simulink library "Solver_DS_SF"  (Simulink 7.1)
libraries: simulink x65
(part 2 of 2)

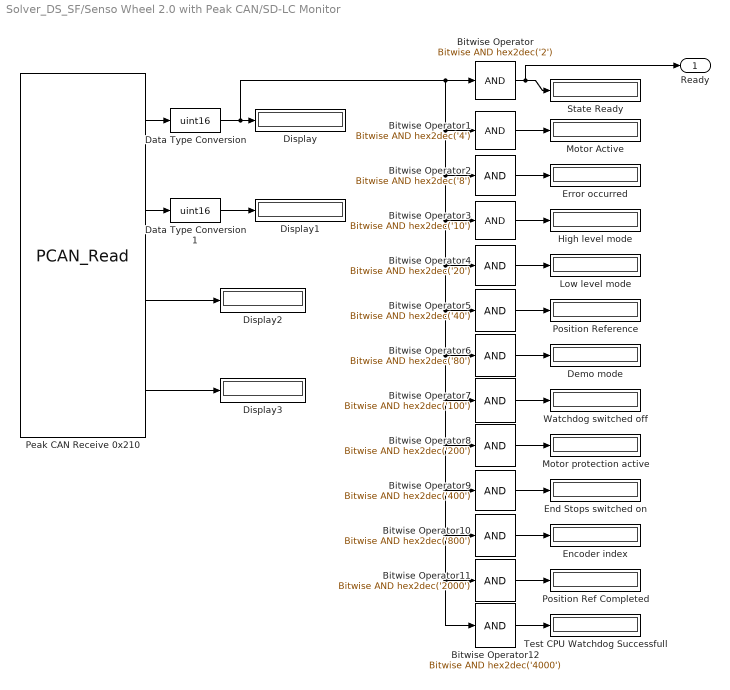
== system Solver_DS_SF/Senso Wheel 2.0 with Peak CAN/SD-LC Monitor ==
  Bitwise Operator : simulink/Logic and Bit Operations/Bitwise Operator  logicop=AND  UseBitMask=on  BitMask=hex2dec('2')  BitMaskRealWorld=Stored Integer
  Bitwise Operator1 : simulink/Logic and Bit Operations/Bitwise Operator  logicop=AND  UseBitMask=on  BitMask=hex2dec('4')  BitMaskRealWorld=Stored Integer
  Bitwise Operator10 : simulink/Logic and Bit Operations/Bitwise Operator  logicop=AND  UseBitMask=on  BitMask=hex2dec('800')  BitMaskRealWorld=Stored Integer
  Bitwise Operator11 : simulink/Logic and Bit Operations/Bitwise Operator  logicop=AND  UseBitMask=on  BitMask=hex2dec('2000')  BitMaskRealWorld=Stored Integer
  Bitwise Operator12 : simulink/Logic and Bit Operations/Bitwise Operator  logicop=AND  UseBitMask=on  BitMask=hex2dec('4000')  BitMaskRealWorld=Stored Integer
  Bitwise Operator2 : simulink/Logic and Bit Operations/Bitwise Operator  logicop=AND  UseBitMask=on  BitMask=hex2dec('8')  BitMaskRealWorld=Stored Integer
  Bitwise Operator3 : simulink/Logic and Bit Operations/Bitwise Operator  logicop=AND  UseBitMask=on  BitMask=hex2dec('10')  BitMaskRealWorld=Stored Integer
  Bitwise Operator4 : simulink/Logic and Bit Operations/Bitwise Operator  logicop=AND  UseBitMask=on  BitMask=hex2dec('20')  BitMaskRealWorld=Stored Integer
  Bitwise Operator5 : simulink/Logic and Bit Operations/Bitwise Operator  logicop=AND  UseBitMask=on  BitMask=hex2dec('40')  BitMaskRealWorld=Stored Integer
  Bitwise Operator6 : simulink/Logic and Bit Operations/Bitwise Operator  logicop=AND  UseBitMask=on  BitMask=hex2dec('80')  BitMaskRealWorld=Stored Integer
  Bitwise Operator7 : simulink/Logic and Bit Operations/Bitwise Operator  logicop=AND  UseBitMask=on  BitMask=hex2dec('100')  BitMaskRealWorld=Stored Integer
  Bitwise Operator8 : simulink/Logic and Bit Operations/Bitwise Operator  logicop=AND  UseBitMask=on  BitMask=hex2dec('200')  BitMaskRealWorld=Stored Integer
  Bitwise Operator9 : simulink/Logic and Bit Operations/Bitwise Operator  logicop=AND  UseBitMask=on  BitMask=hex2dec('400')  BitMaskRealWorld=Stored Integer
  Data Type Conversion : DataTypeConversion  OutDataTypeStr=uint16  OutDataTypeMode=uint16  RndMeth=Zero
  Data Type Conversion1 : DataTypeConversion  OutDataTypeStr=uint16  OutDataTypeMode=uint16  RndMeth=Zero
  Demo mode : Display
  Display{,1..3} (4 alike) : Display
  Encoder index : Display
  End Stops switched on : Display
  Error occurred : Display
  High level mode : Display
  Low level mode : Display
  Motor Active : Display
  Motor protection active : Display
  Peak CAN Receive 0x210 : S-Function  FunctionName=PCAN_Read  Parameters=id,TimeStep,nOut,bits_define  EnableBusSupport=off  mask{id=528, TimeStep=0.1, bits_define={[0:15],[16:31],[32:47],[48:63]}, portnames={'Status','Errors','End Stop Position','Encodeer Index Position'}}
      mask prompts: id "CAN ID"; TimeStep "Sample time"; bits_define "Bit defination (cell array):"; portnames "Port name (cell array):"
      mask init:
      | nOut=length(bits_define);
      | [bits_define]=formatbit(bits_define,portnames,1);
      | set_param(gcb, 'Parameters', ['id,TimeStep,nOut,bits_define']);
      mask Display: port_label('output',1,'Status ');port_label('output',2,'Errors ');port_label('output',3,'End Stop Position ');port_label('output',4,'Encodeer Index Position ');
  Position Ref Completed : Display
  Position Reference : Display
  State Ready : Display
  Test CPU Watchdog Successfull : Display
  Watchdog switched off : Display
  Ready : Outport  InitialOutput=0
  wires:
  Data Type Conversion/1 -> Display/1, Bitwise Operator7/1, Bitwise Operator8/1, Bitwise Operator9/1, Bitwise Operator10/1, Bitwise Operator11/1, Bitwise Operator12/1, Bitwise Operator6/1, Bitwise Operator5/1, Bitwise Operator4/1, Bitwise Operator3/1, Bitwise Operator2/1, Bitwise Operator1/1, Bitwise Operator/1
  Bitwise Operator12/1 -> Test CPU Watchdog Successfull/1
  Bitwise Operator11/1 -> Position Ref Completed/1
  Bitwise Operator10/1 -> Encoder index/1
  Bitwise Operator9/1 -> End Stops switched on/1
  Bitwise Operator8/1 -> Motor protection active/1
  Bitwise Operator7/1 -> Watchdog switched off/1
  Bitwise Operator6/1 -> Demo mode/1
  Bitwise Operator5/1 -> Position Reference/1
  Bitwise Operator4/1 -> Low level mode/1
  Bitwise Operator3/1 -> High level mode/1
  Bitwise Operator2/1 -> Error occurred/1
  Bitwise Operator1/1 -> Motor Active/1
  Bitwise Operator/1 -> State Ready/1, Ready/1
  Data Type Conversion1/1 -> Display1/1
  Peak CAN Receive 0x210/4 -> Display3/1
  Peak CAN Receive 0x210/3 -> Display2/1
  Peak CAN Receive 0x210/2 -> Data Type Conversion1/1
  Peak CAN Receive 0x210/1 -> Data Type Conversion/1

== system Solver_DS_SF/Senso Wheel 2.0 with Peak CAN/Triggered Subsystem ==
  Trigger : TriggerPort
  Constant3 : Constant  OutDataTypeStr=uint8  OutDataTypeMode=uint8
  Ready : Outport  InitialOutput=0
  wires:
  Constant3/1 -> Ready/1

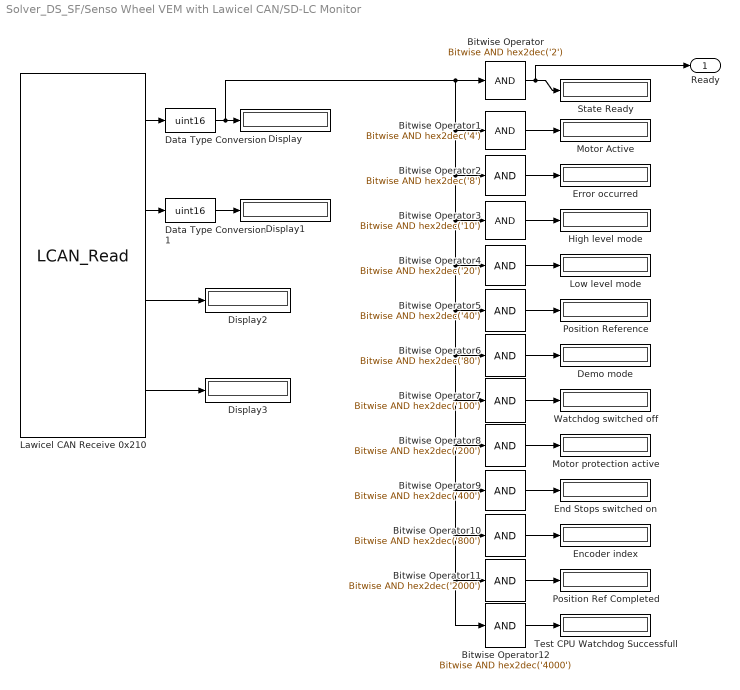
== system Solver_DS_SF/Senso Wheel VEM with Lawicel CAN/SD-LC Monitor ==
  Bitwise Operator : simulink/Logic and Bit Operations/Bitwise Operator  logicop=AND  UseBitMask=on  BitMask=hex2dec('2')  BitMaskRealWorld=Stored Integer
  Bitwise Operator1 : simulink/Logic and Bit Operations/Bitwise Operator  logicop=AND  UseBitMask=on  BitMask=hex2dec('4')  BitMaskRealWorld=Stored Integer
  Bitwise Operator10 : simulink/Logic and Bit Operations/Bitwise Operator  logicop=AND  UseBitMask=on  BitMask=hex2dec('800')  BitMaskRealWorld=Stored Integer
  Bitwise Operator11 : simulink/Logic and Bit Operations/Bitwise Operator  logicop=AND  UseBitMask=on  BitMask=hex2dec('2000')  BitMaskRealWorld=Stored Integer
  Bitwise Operator12 : simulink/Logic and Bit Operations/Bitwise Operator  logicop=AND  UseBitMask=on  BitMask=hex2dec('4000')  BitMaskRealWorld=Stored Integer
  Bitwise Operator2 : simulink/Logic and Bit Operations/Bitwise Operator  logicop=AND  UseBitMask=on  BitMask=hex2dec('8')  BitMaskRealWorld=Stored Integer
  Bitwise Operator3 : simulink/Logic and Bit Operations/Bitwise Operator  logicop=AND  UseBitMask=on  BitMask=hex2dec('10')  BitMaskRealWorld=Stored Integer
  Bitwise Operator4 : simulink/Logic and Bit Operations/Bitwise Operator  logicop=AND  UseBitMask=on  BitMask=hex2dec('20')  BitMaskRealWorld=Stored Integer
  Bitwise Operator5 : simulink/Logic and Bit Operations/Bitwise Operator  logicop=AND  UseBitMask=on  BitMask=hex2dec('40')  BitMaskRealWorld=Stored Integer
  Bitwise Operator6 : simulink/Logic and Bit Operations/Bitwise Operator  logicop=AND  UseBitMask=on  BitMask=hex2dec('80')  BitMaskRealWorld=Stored Integer
  Bitwise Operator7 : simulink/Logic and Bit Operations/Bitwise Operator  logicop=AND  UseBitMask=on  BitMask=hex2dec('100')  BitMaskRealWorld=Stored Integer
  Bitwise Operator8 : simulink/Logic and Bit Operations/Bitwise Operator  logicop=AND  UseBitMask=on  BitMask=hex2dec('200')  BitMaskRealWorld=Stored Integer
  Bitwise Operator9 : simulink/Logic and Bit Operations/Bitwise Operator  logicop=AND  UseBitMask=on  BitMask=hex2dec('400')  BitMaskRealWorld=Stored Integer
  Data Type Conversion : DataTypeConversion  OutDataTypeStr=uint16  OutDataTypeMode=uint16  RndMeth=Zero
  Data Type Conversion1 : DataTypeConversion  OutDataTypeStr=uint16  OutDataTypeMode=uint16  RndMeth=Zero
  Demo mode : Display
  Display{,1..3} (4 alike) : Display
  Encoder index : Display
  End Stops switched on : Display
  Error occurred : Display
  High level mode : Display
  Lawicel CAN Receive 0x210 : S-Function  FunctionName=LCAN_Read  Parameters=1,CAN_MODE,id,TimeStep,nOut,bits_define  EnableBusSupport=off  mask{adapter=CAN1, CAN_MODE=Standard (11-bit), id=528, TimeStep=0.1, bits_define={[0:15],[16:31],[32:47],[48:63]}, portnames={'Status','Errors','End Stop Position','Encodeer Index Position'}}
      mask prompts: adapter "CAN adapter"; CAN_MODE "CAN identifier range:"; id "CAN ID"; TimeStep "Sample time"; bits_define "Bit defination (cell array):"; portnames "Port name (cell array):"
      mask init:
      | nOut=length(bits_define);
      | [bits_define]=formatbit(bits_define,portnames,1);
      | set_param(gcb, 'Parameters', [adapter(4) ',CAN_MODE,id,TimeStep,nOut,bits_define']);
      mask StyleString: popup(CAN1|CAN2|CAN3|CAN4),popup(Standard (11-bit)|Extended (29-bit)),edit,edit,edit,edit
      mask Display: port_label('output',1,'Status ');port_label('output',2,'Errors ');port_label('output',3,'End Stop Position ');port_label('output',4,'Encodeer Index Position ');
  Low level mode : Display
  Motor Active : Display
  Motor protection active : Display
  Position Ref Completed : Display
  Position Reference : Display
  State Ready : Display
  Test CPU Watchdog Successfull : Display
  Watchdog switched off : Display
  Ready : Outport  InitialOutput=0
  wires:
  Bitwise Operator12/1 -> Test CPU Watchdog Successfull/1
  Bitwise Operator11/1 -> Position Ref Completed/1
  Bitwise Operator10/1 -> Encoder index/1
  Bitwise Operator9/1 -> End Stops switched on/1
  Bitwise Operator8/1 -> Motor protection active/1
  Bitwise Operator7/1 -> Watchdog switched off/1
  Bitwise Operator6/1 -> Demo mode/1
  Bitwise Operator5/1 -> Position Reference/1
  Bitwise Operator4/1 -> Low level mode/1
  Bitwise Operator3/1 -> High level mode/1
  Bitwise Operator2/1 -> Error occurred/1
  Bitwise Operator1/1 -> Motor Active/1
  Bitwise Operator/1 -> State Ready/1, Ready/1
  Data Type Conversion1/1 -> Display1/1
  Data Type Conversion/1 -> Display/1, Bitwise Operator7/1, Bitwise Operator8/1, Bitwise Operator9/1, Bitwise Operator10/1, Bitwise Operator11/1, Bitwise Operator12/1, Bitwise Operator6/1, Bitwise Operator5/1, Bitwise Operator4/1, Bitwise Operator3/1, Bitwise Operator2/1, Bitwise Operator1/1, Bitwise Operator/1
  Lawicel CAN Receive 0x210/4 -> Display3/1
  Lawicel CAN Receive 0x210/3 -> Display2/1
  Lawicel CAN Receive 0x210/2 -> Data Type Conversion1/1
  Lawicel CAN Receive 0x210/1 -> Data Type Conversion/1

== system Solver_DS_SF/Senso Wheel VEM with Lawicel CAN/Triggered Subsystem ==
  Trigger : TriggerPort
  Constant3 : Constant  OutDataTypeStr=uint8  OutDataTypeMode=uint8
  Ready : Outport  InitialOutput=0
  wires:
  Constant3/1 -> Ready/1

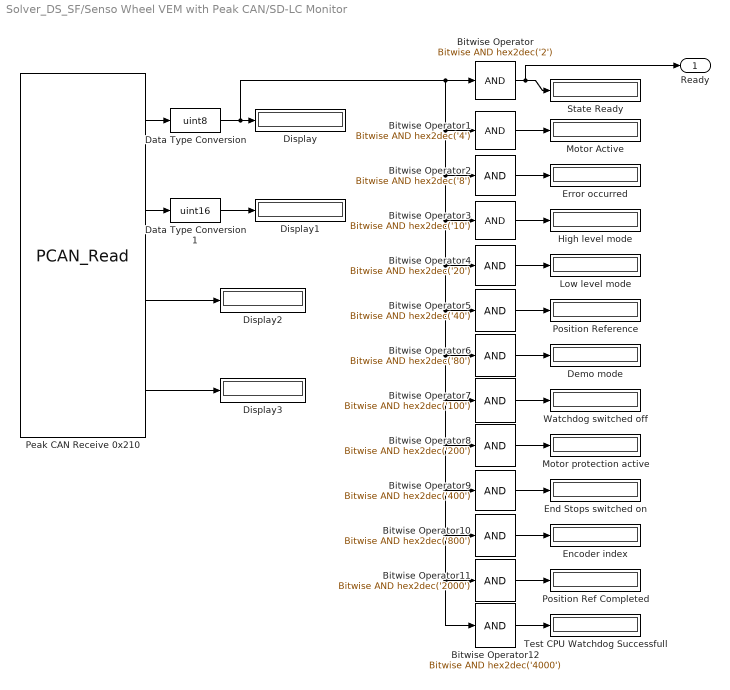
== system Solver_DS_SF/Senso Wheel VEM with Peak CAN/SD-LC Monitor ==
  Bitwise Operator : simulink/Logic and Bit Operations/Bitwise Operator  logicop=AND  UseBitMask=on  BitMask=hex2dec('2')  BitMaskRealWorld=Stored Integer
  Bitwise Operator1 : simulink/Logic and Bit Operations/Bitwise Operator  logicop=AND  UseBitMask=on  BitMask=hex2dec('4')  BitMaskRealWorld=Stored Integer
  Bitwise Operator10 : simulink/Logic and Bit Operations/Bitwise Operator  logicop=AND  UseBitMask=on  BitMask=hex2dec('800')  BitMaskRealWorld=Stored Integer
  Bitwise Operator11 : simulink/Logic and Bit Operations/Bitwise Operator  logicop=AND  UseBitMask=on  BitMask=hex2dec('2000')  BitMaskRealWorld=Stored Integer
  Bitwise Operator12 : simulink/Logic and Bit Operations/Bitwise Operator  logicop=AND  UseBitMask=on  BitMask=hex2dec('4000')  BitMaskRealWorld=Stored Integer
  Bitwise Operator2 : simulink/Logic and Bit Operations/Bitwise Operator  logicop=AND  UseBitMask=on  BitMask=hex2dec('8')  BitMaskRealWorld=Stored Integer
  Bitwise Operator3 : simulink/Logic and Bit Operations/Bitwise Operator  logicop=AND  UseBitMask=on  BitMask=hex2dec('10')  BitMaskRealWorld=Stored Integer
  Bitwise Operator4 : simulink/Logic and Bit Operations/Bitwise Operator  logicop=AND  UseBitMask=on  BitMask=hex2dec('20')  BitMaskRealWorld=Stored Integer
  Bitwise Operator5 : simulink/Logic and Bit Operations/Bitwise Operator  logicop=AND  UseBitMask=on  BitMask=hex2dec('40')  BitMaskRealWorld=Stored Integer
  Bitwise Operator6 : simulink/Logic and Bit Operations/Bitwise Operator  logicop=AND  UseBitMask=on  BitMask=hex2dec('80')  BitMaskRealWorld=Stored Integer
  Bitwise Operator7 : simulink/Logic and Bit Operations/Bitwise Operator  logicop=AND  UseBitMask=on  BitMask=hex2dec('100')  BitMaskRealWorld=Stored Integer
  Bitwise Operator8 : simulink/Logic and Bit Operations/Bitwise Operator  logicop=AND  UseBitMask=on  BitMask=hex2dec('200')  BitMaskRealWorld=Stored Integer
  Bitwise Operator9 : simulink/Logic and Bit Operations/Bitwise Operator  logicop=AND  UseBitMask=on  BitMask=hex2dec('400')  BitMaskRealWorld=Stored Integer
  Data Type Conversion : DataTypeConversion  OutDataTypeStr=uint8  OutDataTypeMode=uint8  RndMeth=Zero
  Data Type Conversion1 : DataTypeConversion  OutDataTypeStr=uint16  OutDataTypeMode=uint16  RndMeth=Zero
  Demo mode : Display
  Display{,1..3} (4 alike) : Display
  Encoder index : Display
  End Stops switched on : Display
  Error occurred : Display
  High level mode : Display
  Low level mode : Display
  Motor Active : Display
  Motor protection active : Display
  Peak CAN Receive 0x210 : S-Function  FunctionName=PCAN_Read  Parameters=id,TimeStep,nOut,bits_define  EnableBusSupport=off  mask{id=528, TimeStep=0.1, bits_define={[0:15],[16:31],[32:47],[48:63]}, portnames={'Status','Errors','End Stop Position','Encodeer Index Position'}}
      mask prompts: id "CAN ID"; TimeStep "Sample time"; bits_define "Bit defination (cell array):"; portnames "Port name (cell array):"
      mask init:
      | nOut=length(bits_define);
      | [bits_define]=formatbit(bits_define,portnames,1);
      | set_param(gcb, 'Parameters', ['id,TimeStep,nOut,bits_define']);
      mask Display: port_label('output',1,'Status ');port_label('output',2,'Errors ');port_label('output',3,'End Stop Position ');port_label('output',4,'Encodeer Index Position ');
  Position Ref Completed : Display
  Position Reference : Display
  State Ready : Display
  Test CPU Watchdog Successfull : Display
  Watchdog switched off : Display
  Ready : Outport  InitialOutput=0
  wires:
  Data Type Conversion/1 -> Display/1, Bitwise Operator7/1, Bitwise Operator8/1, Bitwise Operator9/1, Bitwise Operator10/1, Bitwise Operator11/1, Bitwise Operator12/1, Bitwise Operator6/1, Bitwise Operator5/1, Bitwise Operator4/1, Bitwise Operator3/1, Bitwise Operator2/1, Bitwise Operator1/1, Bitwise Operator/1
  Bitwise Operator12/1 -> Test CPU Watchdog Successfull/1
  Bitwise Operator11/1 -> Position Ref Completed/1
  Bitwise Operator10/1 -> Encoder index/1
  Bitwise Operator9/1 -> End Stops switched on/1
  Bitwise Operator8/1 -> Motor protection active/1
  Bitwise Operator7/1 -> Watchdog switched off/1
  Bitwise Operator6/1 -> Demo mode/1
  Bitwise Operator5/1 -> Position Reference/1
  Bitwise Operator4/1 -> Low level mode/1
  Bitwise Operator3/1 -> High level mode/1
  Bitwise Operator2/1 -> Error occurred/1
  Bitwise Operator1/1 -> Motor Active/1
  Bitwise Operator/1 -> State Ready/1, Ready/1
  Data Type Conversion1/1 -> Display1/1
  Peak CAN Receive 0x210/4 -> Display3/1
  Peak CAN Receive 0x210/3 -> Display2/1
  Peak CAN Receive 0x210/2 -> Data Type Conversion1/1
  Peak CAN Receive 0x210/1 -> Data Type Conversion/1

== system Solver_DS_SF/Senso Wheel VEM with Peak CAN/Triggered Subsystem ==
  Trigger : TriggerPort
  Constant3 : Constant  OutDataTypeStr=uint16  OutDataTypeMode=uint16
  Ready : Outport  InitialOutput=0
  wires:
  Constant3/1 -> Ready/1
